simulink library "INT_EngReq_FullLdIncr"  (R2016b)
settings: Solver=VariableStepAuto  StartTime=0.0  StopTime=10.0  RelTol=1e-3
settings Model: Creator=Administrator  LastModifiedBy=Administrator

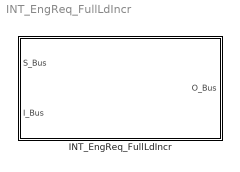
== system INT_EngReq_FullLdIncr ==
  INT_EngReq_FullLdIncr : Subsystem

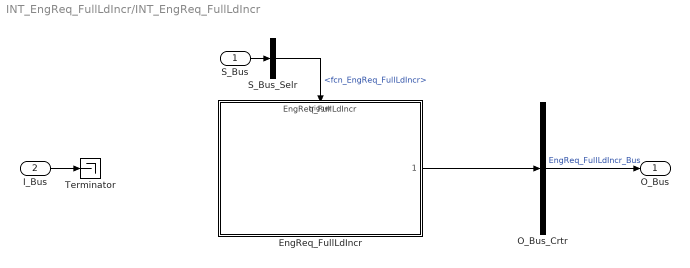
== system INT_EngReq_FullLdIncr/INT_EngReq_FullLdIncr ==
  S_Bus : Inport
  I_Bus : Inport  Port=2
  EngReq_FullLdIncr : ModelReference  ModelNameDialog=EngReq_FullLdIncr  SimulationMode=Normal  ModelReferenceVersion=1.5  TriggerPortName=function  TriggerPortTriggerType=function-call  TriggerPortStatesWhenEnabling=held
  O_Bus_Crtr : BusCreator  Inputs=1
  S_Bus_Selr : BusSelector  OutputSignals=fcn_EngReq_FullLdIncr
  Terminator : Terminator
  O_Bus : Outport
  wires:
  S_Bus_Selr/1 -> EngReq_FullLdIncr/Trigger  "<fcn_EngReq_FullLdIncr>"
  S_Bus/1 -> S_Bus_Selr/1
  I_Bus/1 -> Terminator/1
  O_Bus_Crtr/1 -> O_Bus/1  "EngReq_FullLdIncr_Bus"
  EngReq_FullLdIncr/1 -> O_Bus_Crtr/1
